simulink model "simulator_model"  (Simulink 8.4)
settings: Solver=ode45  StartTime=0.0  StopTime=inf  RelTol=1e-3
values from neighbouring files (symbols this model uses):
  beaver_b = 14.63    [asbdhc2_init.mat]
  beaver_c = 1.5875    [asbdhc2_init.mat]
  beaver_init_p = 0    [asbdhc2_init.mat]
  beaver_init_pitch = 0.13029612885    [asbdhc2_init.mat]
  beaver_init_q = 0    [asbdhc2_init.mat]
  beaver_init_r = 0    [asbdhc2_init.mat]
  beaver_init_roll = 0    [asbdhc2_init.mat]
  beaver_mass = 2288.231    [asbdhc2_init.mat]
  Cl0 = 0.000591    [asbdhc2_init.mat]
  Cl_alpha2_dpt = -0.01406    [asbdhc2_init.mat]
  Cl_beta = -0.0618    [asbdhc2_init.mat]
  Cl_da = -0.09917    [asbdhc2_init.mat]
  Cl_da_alpha = -0.08269    [asbdhc2_init.mat]
  Cl_dr = 0.006934    [asbdhc2_init.mat]
  Cl_p = -0.5045    [asbdhc2_init.mat]
  Cl_r = 0.1695    [asbdhc2_init.mat]
  Cm0 = 0.09448    [asbdhc2_init.mat]
  Cm_alpha = -0.6028    [asbdhc2_init.mat]
  Cm_alpha2 = -2.14    [asbdhc2_init.mat]
  Cm_beta2 = 0.6921    [asbdhc2_init.mat]
  Cm_de = -1.921    [asbdhc2_init.mat]
  Cm_df = 0.4072    [asbdhc2_init.mat]
  Cm_dpt = -0.07895    [asbdhc2_init.mat]
  Cm_q = -15.56    [asbdhc2_init.mat]
  Cm_r = -0.3118    [asbdhc2_init.mat]
  Cn0 = -0.003117    [asbdhc2_init.mat]
  Cn_beta = 0.006719    [asbdhc2_init.mat]
  Cn_beta3 = 0.1373    [asbdhc2_init.mat]
  Cn_da = -0.003872    [asbdhc2_init.mat]
  Cn_dpt3 = -0.003026    [asbdhc2_init.mat]
  Cn_dr = -0.08265    [asbdhc2_init.mat]
  Cn_p = -0.1585    [asbdhc2_init.mat]
  Cn_q = 0.1595    [asbdhc2_init.mat]
  Cn_r = -0.1112    [asbdhc2_init.mat]
  Cx0 = -0.03554    [asbdhc2_init.mat]
  Cx_alpha = 0.00292    [asbdhc2_init.mat]
  Cx_alpha2 = 5.459    [asbdhc2_init.mat]
  Cx_alpha3 = -5.162    [asbdhc2_init.mat]
  Cx_df = -0.09447    [asbdhc2_init.mat]
  Cx_df_alpha = 1.106    [asbdhc2_init.mat]
  Cx_dpt = 0.1161    [asbdhc2_init.mat]
  Cx_dpt2_alpha = 0.1453    [asbdhc2_init.mat]
  Cx_dr = 0.03412    [asbdhc2_init.mat]
  Cx_q = -0.6748    [asbdhc2_init.mat]
  Cy0 = -0.002226    [asbdhc2_init.mat]
  Cy_beta = -0.7678    [asbdhc2_init.mat]
  Cy_da = -0.02956    [asbdhc2_init.mat]
  Cy_dr = 0.1158    [asbdhc2_init.mat]
  Cy_dr_alpha = 0.5238    [asbdhc2_init.mat]
  Cy_p = -0.124    [asbdhc2_init.mat]
  Cy_r = 0.3666    [asbdhc2_init.mat]
  Cz0 = -0.05504    [asbdhc2_init.mat]
  Cz_alpha = -5.578    [asbdhc2_init.mat]
  Cz_alpha3 = 3.442    [asbdhc2_init.mat]
  Cz_de = -0.398    [asbdhc2_init.mat]
  Cz_de_beta = -15.93    [asbdhc2_init.mat]
  Cz_df = -1.377    [asbdhc2_init.mat]
  Cz_df_alpha = -1.261    [asbdhc2_init.mat]
  Cz_dpt = -0.1563    [asbdhc2_init.mat]
  Cz_q = -2.988    [asbdhc2_init.mat]
  uaero0 = [-0.0317656979071 -0.0320210159663 -0.0365180369264 0]    [asbdhc2_init.mat]
undefined symbols (not defined in the file or in its folder): Earth, F, Light, MIL, sigbuilder_block, WGS84
libraries: vrlib x8, aerolibtransform2 x5, aerolibconvert2 x4, aerolibwind2 x3, aerolibfltsims x2, aerolibasang x2, aerolibanimutils x1, aerolibatmos2 x1, aerolibgravity2 x1, aerolib6dof2 x1, aerolibadyn x1
settings Model: Creator=AMANALLAH  LastModifiedBy=AMANALLAH
settings DataIOCC: SignalLoggingSaveFormat=Dataset
settings OptimizationCC: ExpressionDepthLimit=128
settings DebuggingCC: UnderspecifiedInitializationDetection=Simplified  MergeDetectMultiDrivingBlocksExec=error  FcnCallInpInsideContextMsg=EnableAllAsError  StateNameClashWarn=none
settings GRTTargetCC: CombineOutputUpdateFcns=on  GRTInterface=off

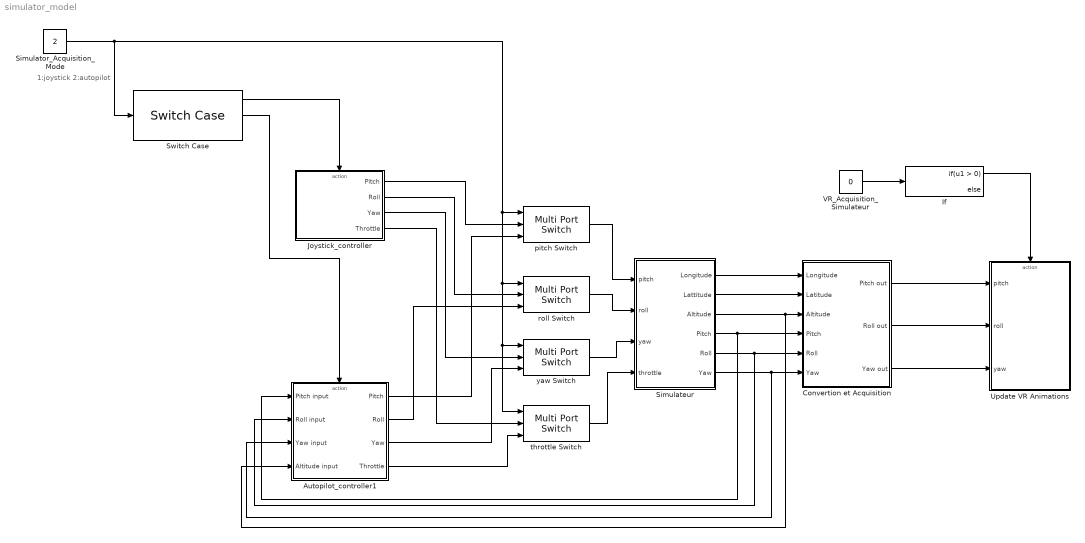
== system simulator_model ==
  note: 1:joystick
      | 2:autopilot
  Autopilot_controller1 : Subsystem  TreatAsAtomicUnit=on
  Convertion et Acquisition : Subsystem
  If : If  SampleTime=0.1
  Joystick_controller : Subsystem  TreatAsAtomicUnit=on
  Simulateur : Subsystem
  Simulator_Acquisition_Mode : Constant  Value=2
  Switch Case : SwitchCase  CaseConditions={1,2}  SampleTime=1/30
  Update VR Animations : Subsystem  TreatAsAtomicUnit=on
  VR_Acquisition_Simulateur : Constant  Value=0
  pitch Switch : MultiPortSwitch  Inputs=2
  roll Switch : MultiPortSwitch  Inputs=2
  throttle Switch : MultiPortSwitch  Inputs=2
  yaw Switch : MultiPortSwitch  Inputs=2
  wires:
  Simulateur/1(Longitude) -> Convertion et Acquisition/1(Longitude)
  Simulateur/2(Lattitude) -> Convertion et Acquisition/2(Latitude)
  Simulateur/3(Altitude) -> Autopilot_controller1/4(Altitude input), Convertion et Acquisition/3(Altitude)
  Simulateur/4(Pitch) -> Autopilot_controller1/1(Pitch input), Convertion et Acquisition/4(Pitch)
  Simulateur/5(Roll) -> Autopilot_controller1/2(Roll input), Convertion et Acquisition/5(Roll)
  Simulateur/6(Yaw) -> Autopilot_controller1/3(Yaw input), Convertion et Acquisition/6(Yaw)
  Convertion et Acquisition/1(Pitch out) -> Update VR Animations/1(pitch)
  Convertion et Acquisition/2(Roll out) -> Update VR Animations/2(roll)
  Convertion et Acquisition/3(Yaw out) -> Update VR Animations/3(yaw)
  pitch Switch/1 -> Simulateur/1(pitch)
  roll Switch/1 -> Simulateur/2(roll)
  yaw Switch/1 -> Simulateur/3(yaw)
  throttle Switch/1 -> Simulateur/4(throttle)
  Autopilot_controller1/1(Pitch) -> pitch Switch/3
  Joystick_controller/1(Pitch) -> pitch Switch/2
  Autopilot_controller1/2(Roll) -> roll Switch/3
  Joystick_controller/2(Roll) -> roll Switch/2
  Joystick_controller/3(Yaw) -> yaw Switch/2
  Autopilot_controller1/3(Yaw) -> yaw Switch/3
  Joystick_controller/4(Throttle) -> throttle Switch/2
  Simulator_Acquisition_Mode/1 -> throttle Switch/1, yaw Switch/1, roll Switch/1, pitch Switch/1, Switch Case/1
  Switch Case/1 -> Joystick_controller/Action
  If/1 -> Update VR Animations/Action
  VR_Acquisition_Simulateur/1 -> If/1
  Autopilot_controller1/4(Throttle) -> throttle Switch/3
  Switch Case/2 -> Autopilot_controller1/Action

== system simulator_model/Autopilot_controller1 ==
  Pitch input : Inport
  Roll input : Inport  Port=2
  Yaw input : Inport  Port=3
  Altitude input : Inport  Port=4
  Action Port : ActionPort  ActionType=case
  Constant{,1..3} (4 alike) : Constant  Value=0
  Pitch : Outport
  Roll : Outport  Port=2
  Yaw : Outport  Port=3
  Throttle : Outport  Port=4
  wires:
  Constant/1 -> Pitch/1
  Constant1/1 -> Roll/1
  Constant2/1 -> Yaw/1
  Constant3/1 -> Throttle/1

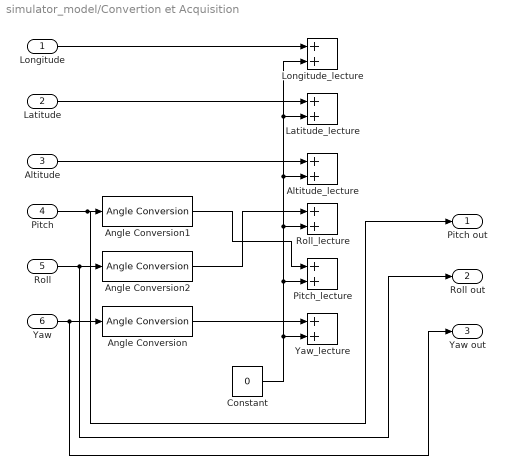
== system simulator_model/Convertion et Acquisition ==
  Longitude : Inport
  Latitude : Inport  Port=2
  Altitude : Inport  Port=3
  Pitch : Inport  Port=4
  Roll : Inport  Port=5
  Yaw : Inport  Port=6
  Altitude_lecture : Sum
  Angle Conversion : aerolibconvert2/Angle Conversion  IU=rad  OU=deg
  Angle Conversion1 : aerolibconvert2/Angle Conversion  IU=rad  OU=deg
  Angle Conversion2 : aerolibconvert2/Angle Conversion  IU=rad  OU=deg
  Constant : Constant  Value=0
  Latitude_lecture : Sum
  Longitude_lecture : Sum
  Pitch_lecture : Sum
  Roll_lecture : Sum
  Yaw_lecture : Sum
  Pitch out : Outport
  Roll out : Outport  Port=2
  Yaw out : Outport  Port=3
  wires:
  Altitude/1 -> Altitude_lecture/1
  Longitude/1 -> Longitude_lecture/1
  Latitude/1 -> Latitude_lecture/1
  Roll/1 -> Angle Conversion2/1, Roll out/1
  Pitch/1 -> Pitch out/1, Angle Conversion1/1
  Constant/1 -> Pitch_lecture/2, Roll_lecture/2, Altitude_lecture/2, Latitude_lecture/2, Longitude_lecture/2, Yaw_lecture/2
  Angle Conversion/1 -> Yaw_lecture/1
  Angle Conversion1/1 -> Pitch_lecture/1
  Angle Conversion2/1 -> Roll_lecture/1
  Yaw/1 -> Angle Conversion/1, Yaw out/1

== system simulator_model/Joystick_controller ==
  Action Port : ActionPort  ActionType=case
  Pilot Joystick : aerolibanimutils/Pilot Joystick  JoystickID=Joystick1  OutputConfiguration=FourAxis  SampleTime=1/30
  Pitch : Outport
  Roll : Outport  Port=2
  Yaw : Outport  Port=3
  Throttle : Outport  Port=4
  wires:
  Pilot Joystick/2 -> Pitch/1
  Pilot Joystick/1 -> Roll/1
  Pilot Joystick/3 -> Yaw/1
  Pilot Joystick/4 -> Throttle/1

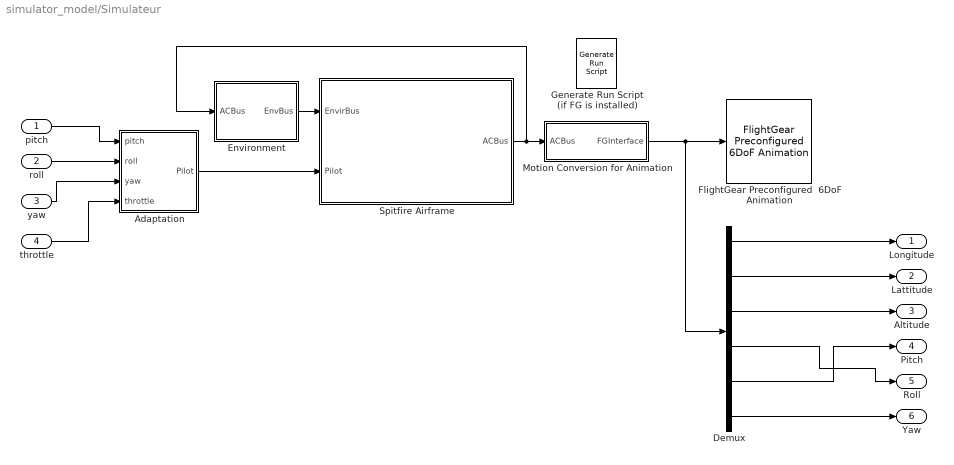
== system simulator_model/Simulateur ==
  pitch : Inport
  roll : Inport  Port=2
  yaw : Inport  Port=3
  throttle : Inport  Port=4
  "Adaptation " : Subsystem
  Demux : Demux  Outputs=6
  Environment : Subsystem
  FlightGear Preconfigured  6DoF Animation : aerolibfltsims/FlightGear Preconfigured 6DoF Animation  xFlightGearVersion=v3.0  DestinationIpAddress=127.0.0.1  DestinationPort=5502  SampleTime=1/30
  Generate Run Script (if FG is installed) : aerolibfltsims/Generate Run Script  OutputFileName=runfg.bat  FlightGearBaseDirectory=C:\Program Files\FlightGear  GeometryModelName=dhc2F  DestinationPort=5502  OriginAddress=127.0.0.1  OriginPort=5505  LocalAddress=127.0.0.1  AirportId=KSFO  RunwayId=10L  InitialAltitude=7224  InitialHeading=113  OffsetDistance=4.72  OffsetAzimuth=0  GenerateFile=off  Architecture=Default  dataFlow=Send
  Motion Conversion for Animation : Subsystem
      mask Display:
      | port_label('input',1,'ACBus')
      | port_label('output',1,'\lambda,L,h,\phi,\theta,\psi','texmode','on')
  Spitfire Airframe : Subsystem
      mask Display: image(imread([pwd,'\Ressources\images\spitfire.jpg']));
  Longitude : Outport
  Lattitude : Outport  Port=2
  Altitude : Outport  Port=3
  Pitch : Outport  Port=4
  Roll : Outport  Port=5
  Yaw : Outport  Port=6
  wires:
  Spitfire Airframe/1(ACBus) -> Motion Conversion for Animation/1(ACBus), Environment/1(ACBus)
  "Adaptation "/1(Pilot) -> Spitfire Airframe/2(Pilot)
  Environment/1(EnvBus) -> Spitfire Airframe/1(EnvirBus)
  Motion Conversion for Animation/1(FGInterface) -> Demux/1, FlightGear Preconfigured  6DoF Animation/1
  pitch/1 -> "Adaptation "/1(pitch)
  roll/1 -> "Adaptation "/2(roll)
  yaw/1 -> "Adaptation "/3(yaw)
  throttle/1 -> "Adaptation "/4(throttle)
  Demux/1 -> Longitude/1
  Demux/2 -> Lattitude/1
  Demux/3 -> Altitude/1
  Demux/4 -> Roll/1
  Demux/5 -> Pitch/1
  Demux/6 -> Yaw/1

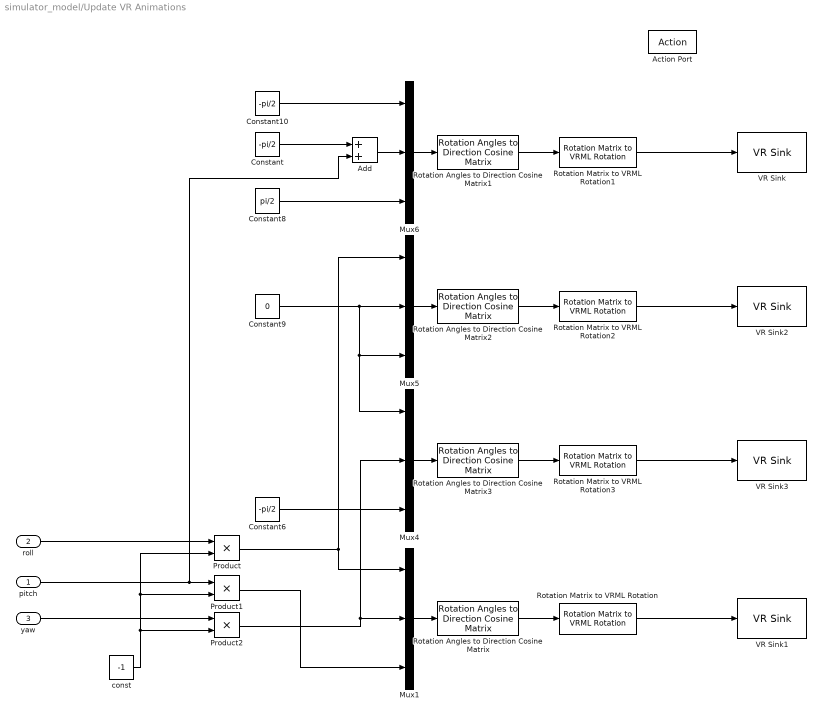
== system simulator_model/Update VR Animations ==
  pitch : Inport
  roll : Inport  Port=2
  yaw : Inport  Port=3
  Action Port : ActionPort  ActionType=then
  Add : Sum
  Constant : Constant  Value=-pi/2
  Constant10 : Constant  Value=-pi/2
  Constant6 : Constant  Value=-pi/2
  Constant8 : Constant  Value=pi/2
  Constant9 : Constant  Value=0
  Mux{1,4..6} (4 alike) : Mux  Inputs=3
  Product : Product
  Product1 : Product
  Product2 : Product
  Rotation Angles to Direction Cosine Matrix{,1..3} (4 alike) : aerolibtransform2/Rotation Angles to Direction Cosine Matrix  rotationOrder=ZYX
  Rotation Matrix to VRML Rotation{,1..3} (4 alike) : vrlib/Utilities/Rotation Matrix to VRML Rotation  maxzero=1e-12
  VR Sink : vrlib/VR Sink  InstantiateOnLoad=on  SampleTime=0.1  ViewEnable=on  RemoteChange=off  RemoteView=off  FieldsWritten=Airplane.rotation.4.1.1.double  WorldFileName=spitfire_3d_pitch.WRL  AutoView=off  VideoDimensions=[]  AllowVariableSize=off
  VR Sink1 : vrlib/VR Sink  InstantiateOnLoad=on  SampleTime=0.1  ViewEnable=on  RemoteChange=off  RemoteView=off  FieldsWritten=Airplane.rotation.4.1.1.double  WorldFileName=spitfire_3d.WRL  AutoView=off  VideoDimensions=[]  AllowVariableSize=off
  VR Sink2 : vrlib/VR Sink  InstantiateOnLoad=on  SampleTime=0.1  ViewEnable=on  RemoteChange=off  RemoteView=off  FieldsWritten=Airplane.rotation.4.1.1.double  WorldFileName=spitfire_3d_roll.WRL  AutoView=off  VideoDimensions=[]  AllowVariableSize=off
  VR Sink3 : vrlib/VR Sink  InstantiateOnLoad=on  SampleTime=0.1  ViewEnable=on  RemoteChange=off  RemoteView=off  FieldsWritten=Airplane.rotation.4.1.1.double  WorldFileName=spitfire_3d_yaw.WRL  AutoView=off  VideoDimensions=[]  AllowVariableSize=off
  const : Constant  Value=-1
  wires:
  Rotation Matrix to VRML Rotation/1 -> VR Sink1/1
  Rotation Angles to Direction Cosine Matrix/1 -> Rotation Matrix to VRML Rotation/1
  Mux1/1 -> Rotation Angles to Direction Cosine Matrix/1
  Mux6/1 -> Rotation Angles to Direction Cosine Matrix1/1
  Rotation Angles to Direction Cosine Matrix1/1 -> Rotation Matrix to VRML Rotation1/1
  Rotation Matrix to VRML Rotation1/1 -> VR Sink/1
  Mux5/1 -> Rotation Angles to Direction Cosine Matrix2/1
  Rotation Angles to Direction Cosine Matrix2/1 -> Rotation Matrix to VRML Rotation2/1
  Rotation Matrix to VRML Rotation2/1 -> VR Sink2/1
  Mux4/1 -> Rotation Angles to Direction Cosine Matrix3/1
  Rotation Angles to Direction Cosine Matrix3/1 -> Rotation Matrix to VRML Rotation3/1
  Rotation Matrix to VRML Rotation3/1 -> VR Sink3/1
  Constant9/1 -> Mux4/1, Mux5/3, Mux5/2
  Constant6/1 -> Mux4/3
  Constant10/1 -> Mux6/1
  Constant8/1 -> Mux6/3
  Constant/1 -> Add/1
  Add/1 -> Mux6/2
  Product/1 -> Mux1/1, Mux5/1
  Product2/1 -> Mux4/2, Mux1/2
  Product1/1 -> Mux1/3
  roll/1 -> Product/1
  pitch/1 -> Product1/1, Add/2
  yaw/1 -> Product2/1
  const/1 -> Product/2, Product1/2, Product2/2

== system simulator_model/Simulateur/Adaptation  ==
  pitch : Inport
  roll : Inport  Port=2
  yaw : Inport  Port=3
  throttle : Inport  Port=4
  Bus Creator : BusCreator  Inputs=2
  Flap : Subsystem  Tag=STV Subsys  LoadFcn=sigbuilder_block('load');  StartFcn=sigbuilder_block('start');  StopFcn=sigbuilder_block('stop');  ClipboardFcn=sigbuilder_block('clipboard');  mask(Sigbuilder block){}
      mask help: Sigbuilder GUI
      mask init:
      | if ~strcmp(get_param(bdroot(gcb),'SimulationStatus'),'stopped') tuvar = sigbuilder_block('maskInit'); end
      settings: CopyFcn=sigbuilder_block('copy');  DeleteFcn=sigbuilder_block('delete');  ModelCloseFcn=sigbuilder_block('modelClose');  PreSaveFcn=sigbuilder_block('preSave');  PauseFcn=sigbuilder_block('pause')  ContinueFcn=sigbuilder_block('continue')  NameChangeFcn=sigbuilder_block('namechange');  OpenFcn=sigbuilder_block('open',[127.2 252 511.2 271.2 ]);  CloseFcn=sigbuilder_block('close');
      mask Display: plot(0,0,100,100,[10,10,40,40,10],[80,20,20,80,80],[40,10],[50,50], [40,27,10],[65,72,56],[40,25,25,10],[28,28,43,43]);
  Input Signal  Conditioning : Subsystem
  Mux2 : Mux  Inputs=3
  Rate Transition1 : RateTransition  OutPortSampleTime=0
  Rate Transition2 : RateTransition  OutPortSampleTime=0
  Pilot : Outport
  wires:
  Flap/1(Flap) -> Input Signal  Conditioning/3(Flap)
  Rate Transition1/1 -> Input Signal  Conditioning/1(Stick / Throt)
  Rate Transition2/1 -> Input Signal  Conditioning/2(Rudder)
  Input Signal  Conditioning/1(uaero) -> Bus Creator/1  "uaero"
  Input Signal  Conditioning/2(uprop) -> Bus Creator/2  "uprop"
  Bus Creator/1 -> Pilot/1
  Mux2/1 -> Rate Transition1/1
  roll/1 -> Mux2/1
  yaw/1 -> Rate Transition2/1
  throttle/1 -> Mux2/3
  pitch/1 -> Mux2/2

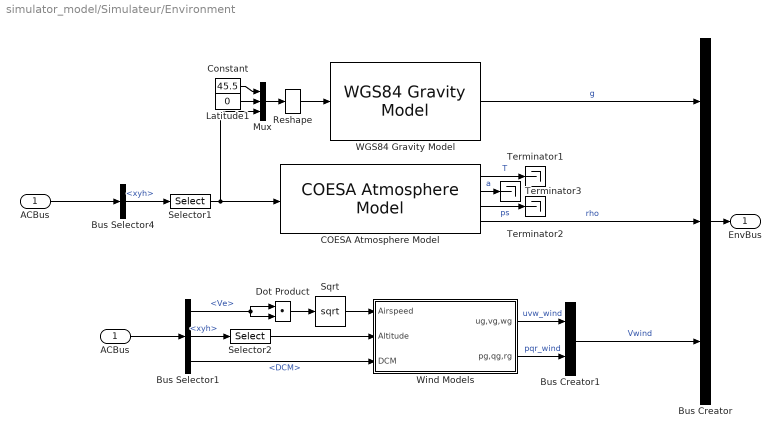
== system simulator_model/Simulateur/Environment ==
  ACBus : Inport
  "ACBus " : InportShadow
  Bus Creator : BusCreator  Inputs=3
  Bus Creator1 : BusCreator  Inputs=2
  Bus Selector1 : BusSelector  OutputSignals=Ve,xyh,DCM
  Bus Selector4 : BusSelector  OutputSignals=xyh
  COESA Atmosphere Model : aerolibatmos2/COESA Atmosphere Model  units=Metric (MKS)  spec=1976 COESA-extended U.S. Standard Atmosphere  model=Profile  profile_var=High temperature  profile_percent=1%  profile_alt=5 km (16404 ft)  envelope_var=High temperature  envelope_percent=1%  action=Warning
  Constant : Constant  Value=45.5
  Dot Product : DotProduct  InputSameDT=on  OutDataTypeStr=Inherit: Inherit via internal rule
  Latitude1 : Constant  Value=0
  Mux : Mux  Inputs=3
  Reshape : Reshape  OutputDimensionality=Row vector (2-D)
  Selector1 : Selector  IndexMode=Zero-based  InputPortWidth=3  Indices=2
  Selector2 : Selector  IndexMode=Zero-based  InputPortWidth=3  Indices=2
  Sqrt : Sqrt  SaturateOnIntegerOverflow=on
  Terminator1 : Terminator
  Terminator2 : Terminator
  Terminator3 : Terminator
  "WGS84 Gravity Model " : aerolibgravity2/WGS84 Gravity Model   model=WGS84 Taylor Series  units=Metric (MKS)  no_atmos=on  precessing=on  jd_loc=off  month=October  day=10  year=2004  no_centrifugal=on  action=None
  Wind Models : Subsystem
  EnvBus : Outport
  wires:
  COESA Atmosphere Model/4 -> Bus Creator/2  "rho"
  COESA Atmosphere Model/1 -> Terminator1/1  "T"
  COESA Atmosphere Model/3 -> Terminator2/1  "ps"
  COESA Atmosphere Model/2 -> Terminator3/1  "a"
  Selector1/1 -> COESA Atmosphere Model/1, Mux/3
  Bus Selector1/3 -> Wind Models/3(DCM)  "<DCM>"
  Wind Models/2(pg,qg,rg) -> Bus Creator1/2  "pqr_wind"
  Wind Models/1(ug,vg,wg) -> Bus Creator1/1  "uvw_wind"
  Bus Creator1/1 -> Bus Creator/3  "Vwind"
  Dot Product/1 -> Sqrt/1
  Sqrt/1 -> Wind Models/1(Airspeed)
  Bus Creator/1 -> EnvBus/1
  ACBus/1 -> Bus Selector4/1
  Bus Selector4/1 -> Selector1/1  "<xyh>"
  "ACBus "/1 -> Bus Selector1/1
  Bus Selector1/2 -> Selector2/1  "<xyh>"
  Selector2/1 -> Wind Models/2(Altitude)
  Bus Selector1/1 -> Dot Product/1, Dot Product/2  "<Ve>"
  Constant/1 -> Mux/1
  Latitude1/1 -> Mux/2
  Mux/1 -> Reshape/1
  "WGS84 Gravity Model "/1 -> Bus Creator/1  "g"
  Reshape/1 -> "WGS84 Gravity Model "/1

== system simulator_model/Simulateur/Motion Conversion for Animation ==
  ACBus : Inport
  Bus Selector : BusSelector  OutputSignals=phi_theta_psi
  Bus Selector1 : BusSelector  OutputSignals=Xe  OutputAsBus=on
  Constant : Constant  Value=0
  Flat Earth to LLA : aerolibtransform2/Flat Earth to LLA  units=Metric (MKS)  ptype=Earth (WGS84)  F=1/298.257223563  R=6378137  LL0=[37.6272 -122.3896]  psi=0
  Mux : Mux  Inputs=2
  Mux1 : Mux  Inputs=2
  Selector : Selector  IndexMode=Zero-based  InputPortWidth=2  Indices=[1 0]
  FGInterface : Outport
  wires:
  Mux1/1 -> FGInterface/1
  Constant/1 -> Flat Earth to LLA/2
  Bus Selector/1 -> Mux1/2  "<phi_theta_psi>"
  Mux/1 -> Mux1/1
  Flat Earth to LLA/2 -> Mux/2
  Flat Earth to LLA/1 -> Selector/1
  Bus Selector1/1 -> Flat Earth to LLA/1
  ACBus/1 -> Bus Selector/1, Bus Selector1/1
  Selector/1 -> Mux/1

== system simulator_model/Simulateur/Spitfire Airframe ==
  EnvirBus : Inport
  Pilot : Inport  Port=2
  Aircraft Dynamics : Subsystem
  Calculate Parameters : Subsystem
  ACBus : Outport
  wires:
  Pilot/1 -> Aircraft Dynamics/1(Pilot)
  Aircraft Dynamics/1(AC Bus) -> ACBus/1, Calculate Parameters/2(ACBus)
  EnvirBus/1 -> Aircraft Dynamics/2(EnvirBus), Calculate Parameters/1(EnvirBus)
  Calculate Parameters/1(FltParams) -> Aircraft Dynamics/3(FltParams)

== system simulator_model/Simulateur/Adaptation /Flap ==
  Demux : Demux  Tag=STV Demux  Outputs=1
  FromWs : FromWorkspace  Tag=STV FromWs  VariableName=tuvar  SampleTime=0  OutputAfterFinalValue=Holding final value  SigBuilderData=DataTag0  VnvData=DataTag1
      SigBuilderData=|
      | dataSet.timeRange = [0 300]
      | dataSet.name = 'Group 1'
      | sbobj.Groups.Name = 'Group 1'
      | sbobj.Groups.Signals.Name = 'Flap'
      | sbobj.Groups.Signals.XData = [0 4 6 300]
      | sbobj.Groups.Signals.YData = [0 0 0 0]
      | sbobj.Groups.TimeRange = [0 300]
  Flap : Outport  Tag=STV Outport
  wires:
  Demux/1 -> Flap/1
  FromWs/1 -> Demux/1

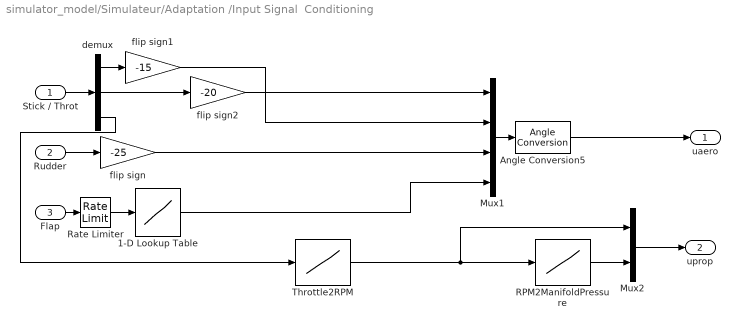
== system simulator_model/Simulateur/Adaptation /Input Signal  Conditioning ==
  Stick / Throt : Inport
  Rudder : Inport  Port=2
  Flap : Inport  Port=3
  1-D Lookup Table : Lookup_n-D  NumberOfTableDimensions=1  BreakpointsForDimension1=[0:3]  Table=[0 4 10 20]  SaturateOnIntegerOverflow=on  InputSameDT=on
  Angle Conversion5 : aerolibconvert2/Angle Conversion  IU=deg  OU=rad
  Mux1 : Mux
  Mux2 : Mux  Inputs=2
  RPM2ManifoldPressure : Lookup_n-D  NumberOfTableDimensions=1  BreakpointsForDimension1=[0 1800 2300]  IndexSearchMethod=Linear search  BeginIndexSearchUsingPreviousIndexResult=on  Table=[0 22.5735 26]  ExtrapMethod=Clip  InputSameDT=on
  Rate Limiter : RateLimiter  RisingSlewLimit=0.5  FallingSlewLimit=-0.5
  Throttle2RPM : Lookup_n-D  NumberOfTableDimensions=1  BreakpointsForDimension1=(1/6)*(3+([-3:3]))  IndexSearchMethod=Linear search  BeginIndexSearchUsingPreviousIndexResult=on  Table=((1+tanh([-3:3]))/(1+tanh(2.65))-0.0025)*2300  ExtrapMethod=Clip  InputSameDT=on
  demux : Demux  Outputs=3
  flip sign : Gain  Gain=-25  SaturateOnIntegerOverflow=on  OutDataTypeStr=Inherit: Same as input  ParamDataTypeStr=Inherit: Same as input
  flip sign1 : Gain  Gain=-15  SaturateOnIntegerOverflow=on  OutDataTypeStr=Inherit: Same as input  ParamDataTypeStr=Inherit: Same as input
  flip sign2 : Gain  Gain=-20  SaturateOnIntegerOverflow=on  OutDataTypeStr=Inherit: Same as input  ParamDataTypeStr=Inherit: Same as input
  uaero : Outport
  uprop : Outport  Port=2
  wires:
  demux/3 -> Throttle2RPM/1
  Flap/1 -> Rate Limiter/1
  Rate Limiter/1 -> 1-D Lookup Table/1
  Stick / Throt/1 -> demux/1
  Rudder/1 -> flip sign/1
  1-D Lookup Table/1 -> Mux1/4
  demux/1 -> flip sign1/1
  demux/2 -> flip sign2/1
  Mux1/1 -> Angle Conversion5/1
  Angle Conversion5/1 -> uaero/1
  RPM2ManifoldPressure/1 -> Mux2/2
  Mux2/1 -> uprop/1
  flip sign/1 -> Mux1/3
  Throttle2RPM/1 -> Mux2/1, RPM2ManifoldPressure/1
  flip sign1/1 -> Mux1/2
  flip sign2/1 -> Mux1/1

== system simulator_model/Simulateur/Environment/Wind Models ==
  Airspeed : Inport
  Altitude : Inport  Port=2
  DCM : Inport  Port=3
  "DCM " : InportShadow  Port=3
  Discrete Wind Gust Model : aerolibwind2/Discrete Wind Gust Model  units=Metric (MKS)  Gx=off  Gy=off  Gz=off  t_0=20  d_m=[120 120 80]  v_m=[3.5 3.5 3.0]
  Dryden Wind Turbulence Model  (Continuous (+q -r)) : aerolibwind2/Dryden Wind Turbulence Model  (Continuous (+q -r))  units=Metric (MKS)  spec=MIL-F-8785C  model=Continuous Dryden (+q -r)  W20=5  Wdeg=0  TurbProb=10^-2 - Light  L_high=533.4  Wingspan=4  ts=0.1  Seed=[23341 23342 23343 23344]  T_on=off
  Sum : Sum  Inputs=+++  SaturateOnIntegerOverflow=on  InputSameDT=on  OutDataTypeStr=Inherit: Same as first input
  Wind Shear Model : aerolibwind2/Wind Shear Model  units=Metric (MKS)  phase=Category C - Terminal Flight Phase  W_20=0  Wdeg=0
  ug,vg,wg : Outport
  pg,qg,rg : Outport  Port=2
  wires:
  "DCM "/1 -> Dryden Wind Turbulence Model  (Continuous (+q -r))/3
  Wind Shear Model/1 -> Sum/1
  Dryden Wind Turbulence Model  (Continuous (+q -r))/1 -> Sum/2
  Discrete Wind Gust Model/1 -> Sum/3
  Sum/1 -> ug,vg,wg/1
  DCM/1 -> Wind Shear Model/2
  Airspeed/1 -> Dryden Wind Turbulence Model  (Continuous (+q -r))/2, Discrete Wind Gust Model/1
  Dryden Wind Turbulence Model  (Continuous (+q -r))/2 -> pg,qg,rg/1
  Altitude/1 -> Dryden Wind Turbulence Model  (Continuous (+q -r))/1, Wind Shear Model/1

== system simulator_model/Simulateur/Spitfire Airframe/Aircraft Dynamics ==
  Pilot : Inport
  EnvirBus : Inport  Port=2
  FltParams : Inport  Port=3
  6DOF (Quaternion) : aerolib6dof2/6DOF (Euler Angles)  units=Metric (MKS)  mtype=Fixed  rep=Quaternion  xme_0=xme_0  Vm_0=[44.54 2.714 5.836]  eul_0=[beaver_init_roll, beaver_init_pitch, 113/180*pi]  pm_0=[beaver_init_p, beaver_init_q, beaver_init_r]  mass_0=beaver_mass  mass_e=0  mass_f=0  inertia="[5.787969e3  0 1.1764e2; 0 6.92893e3 0; -1.1764e2 0 1.1578329e4]"  inertia_e=eye(3)  inertia_f=eye(3)  k_quat=1.0  vre_flag=on
  Bus Creator : BusCreator  Inputs=8
  Hdot : Gain  Gain=-1  SaturateOnIntegerOverflow=on  OutDataTypeStr=Inherit: Same as input  ParamDataTypeStr=Inherit: Same as input
  Selector1 : Selector  IndexMode=Zero-based  InputPortWidth=3  Indices=2
  Terminator : Terminator
  Terminator1 : Terminator
  Total Forces  and Moments : Subsystem
  xyH : Gain  Gain=[1 1 -1]  SaturateOnIntegerOverflow=on  OutDataTypeStr=Inherit: Same as input  ParamDataTypeStr=Inherit: Same as input
  AC Bus : Outport
  wires:
  6DOF (Quaternion)/4 -> Bus Creator/6, Total Forces  and Moments/3(DCM)  "DCM"
  6DOF (Quaternion)/3 -> Bus Creator/5  "phi_theta_psi"
  6DOF (Quaternion)/2 -> xyH/1, Bus Creator/3  "Xe"
  6DOF (Quaternion)/5 -> Bus Creator/7  "Vbody"
  6DOF (Quaternion)/7 -> Terminator/1
  6DOF (Quaternion)/1 -> Selector1/1, Bus Creator/2  "Ve"
  Pilot/1 -> Total Forces  and Moments/2(Pilot)
  Selector1/1 -> Hdot/1
  Total Forces  and Moments/1(Total Force) -> 6DOF (Quaternion)/1
  Total Forces  and Moments/2(Total Moment) -> 6DOF (Quaternion)/2
  xyH/1 -> Bus Creator/4  "xyh"
  Hdot/1 -> Bus Creator/1  "Hdot"
  6DOF (Quaternion)/8 -> Terminator1/1
  Bus Creator/1 -> AC Bus/1
  EnvirBus/1 -> Total Forces  and Moments/1(EnvirBus)
  6DOF (Quaternion)/6 -> Bus Creator/8  "pqr"
  FltParams/1 -> Total Forces  and Moments/4(FltParams)

== system simulator_model/Simulateur/Spitfire Airframe/Calculate Parameters ==
  EnvirBus : Inport
  ACBus : Inport  Port=2
  "ACBus " : InportShadow  Port=2
  Bus Creator : BusCreator  Inputs=5
  Bus Selector1 : BusSelector  OutputSignals=rho
  Bus Selector2 : BusSelector  OutputSignals=Vbody
  Bus Selector3 : BusSelector  OutputSignals=pqr,Ve
  Bus Selector4 : BusSelector  OutputSignals=Vwind.uvw_wind,Vwind.pqr_wind
  Dynamic Pressure : aerolibasang/Dynamic Pressure
  "Incidence, Sideslip, & Airspeed" : aerolibasang/Incidence, Sideslip, & Airspeed
  Sum2 : Sum  Inputs=|++  SaturateOnIntegerOverflow=on  InputSameDT=on  OutDataTypeStr=Inherit: Same as first input
  Sum4 : Sum  Inputs=+-|  SaturateOnIntegerOverflow=on  InputSameDT=on  OutDataTypeStr=Inherit: Same as first input
  FltParams : Outport
  wires:
  "ACBus "/1 -> Bus Selector2/1
  Bus Creator/1 -> FltParams/1
  Bus Selector3/1 -> Sum2/2  "<pqr>"
  ACBus/1 -> Bus Selector3/1
  Bus Selector1/1 -> Dynamic Pressure/2  "<rho>"
  EnvirBus/1 -> Bus Selector1/1, Bus Selector4/1
  Dynamic Pressure/1 -> Bus Creator/5  "Qdyn"
  Bus Selector3/2 -> Dynamic Pressure/1  "<Ve>"
  Bus Selector4/2 -> Sum2/1  "<pqr_wind>"
  Sum4/1 -> "Incidence, Sideslip, & Airspeed"/1
  "Incidence, Sideslip, & Airspeed"/1 -> Bus Creator/1  "alpha"
  "Incidence, Sideslip, & Airspeed"/2 -> Bus Creator/2  "beta"
  "Incidence, Sideslip, & Airspeed"/3 -> Bus Creator/3  "V"
  Bus Selector2/1 -> Sum4/1  "<Vbody>"
  Bus Selector4/1 -> Sum4/2  "<uvw_wind>"
  Sum2/1 -> Bus Creator/4  "pqr_tot"

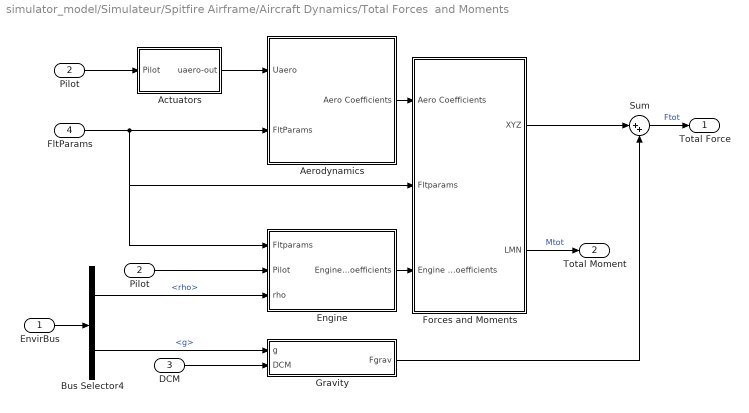
== system simulator_model/Simulateur/Spitfire Airframe/Aircraft Dynamics/Total Forces  and Moments ==
  EnvirBus : Inport
  Pilot : Inport  Port=2
  DCM : Inport  Port=3
  FltParams : Inport  Port=4
  Actuators : Subsystem
  Aerodynamics : Subsystem
  Bus Selector4 : BusSelector  OutputSignals=rho,g
  "Engine " : Subsystem
  Forces and Moments : Subsystem
  "Gravity " : Subsystem
  "Pilot " : InportShadow  Port=2
  Sum : Sum  Inputs=|++  SaturateOnIntegerOverflow=on  InputSameDT=on  OutDataTypeStr=Inherit: Same as first input
  Total Force : Outport
  Total Moment : Outport  Port=2
  wires:
  Forces and Moments/1(XYZ) -> Sum/1
  "Engine "/1(Engine Coefficients) -> Forces and Moments/3(Engine Coefficients)
  "Gravity "/1(Fgrav) -> Sum/2
  Aerodynamics/1(Aero Coefficients) -> Forces and Moments/1(Aero Coefficients)
  Pilot/1 -> Actuators/1(Pilot)
  Bus Selector4/1 -> "Engine "/3(rho)  "<rho>"
  DCM/1 -> "Gravity "/2(DCM)
  Bus Selector4/2 -> "Gravity "/1(g)  "<g>"
  Sum/1 -> Total Force/1  "Ftot"
  Forces and Moments/2(LMN) -> Total Moment/1  "Mtot"
  "Pilot "/1 -> "Engine "/2(Pilot)
  FltParams/1 -> "Engine "/1(Fltparams), Forces and Moments/2(Fltparams), Aerodynamics/2(FltParams)
  Actuators/1(uaero-out) -> Aerodynamics/1(Uaero)
  EnvirBus/1 -> Bus Selector4/1

== system simulator_model/Simulateur/Spitfire Airframe/Aircraft Dynamics/Total Forces  and Moments/Actuators ==
  Pilot : Inport
  Bus Selector2 : BusSelector  OutputSignals=uaero
  Demux : Demux
  Initial inputs for aero : Constant  Value=uaero0
  Mux : Mux
  Sum1 : Sum  Inputs=++|  SaturateOnIntegerOverflow=on  InputSameDT=on  OutDataTypeStr=Inherit: Same as first input
  uaero-out : Outport
  wires:
  Pilot/1 -> Bus Selector2/1
  Initial inputs for aero/1 -> Sum1/1
  Sum1/1 -> uaero-out/1
  Bus Selector2/1 -> Demux/1  "<uaero>"
  Demux/4 -> Mux/4
  Demux/1 -> Mux/1
  Demux/2 -> Mux/2
  Demux/3 -> Mux/3
  Mux/1 -> Sum1/2

== system simulator_model/Simulateur/Spitfire Airframe/Aircraft Dynamics/Total Forces  and Moments/Aerodynamics ==
  Uaero : Inport
  FltParams : Inport  Port=2
  Actuator Increments : Subsystem
  Body Rate Damping : Subsystem
  Bus Selector1 : BusSelector  OutputSignals=alpha,beta
  Bus Selector2 : BusSelector  OutputSignals=V,pqr_tot
  Datum Coefficients : Subsystem
  Sum : Sum  Inputs=+++  SaturateOnIntegerOverflow=on
  Aero Coefficients : Outport
  wires:
  Bus Selector1/2 -> Actuator Increments/2(beta), Datum Coefficients/2(beta)  "<beta>"
  Sum/1 -> Aero Coefficients/1
  Body Rate Damping/1(Coefficients) -> Sum/3
  Datum Coefficients/1(Coefficients) -> Sum/1
  Actuator Increments/1(Coefficients) -> Sum/2
  Bus Selector2/1 -> Body Rate Damping/1(V)  "<V>"
  Bus Selector2/2 -> Body Rate Damping/2(p,q,r)  "<pqr_tot>"
  Uaero/1 -> Actuator Increments/3(Actuator Deflections)
  Bus Selector1/1 -> Actuator Increments/1(alpha), Datum Coefficients/1(alpha)  "<alpha>"
  FltParams/1 -> Bus Selector1/1, Bus Selector2/1

== system simulator_model/Simulateur/Spitfire Airframe/Aircraft Dynamics/Total Forces  and Moments/Engine  ==
  Fltparams : Inport
  Pilot : Inport  Port=2
  rho : Inport  Port=3
  Bus Selector4 : BusSelector  OutputSignals=V,alpha
  eng : Subsystem
  pow : Subsystem
  Engine Coefficients : Outport
  wires:
  Bus Selector4/1 -> pow/3(V)  "<V>"
  rho/1 -> pow/1(rho)
  Bus Selector4/2 -> eng/2(alpha)  "<alpha>"
  eng/1(Cprop) -> Engine Coefficients/1
  Pilot/1 -> pow/2(Pilot)
  pow/1(dpt) -> eng/1(dpt)
  Fltparams/1 -> Bus Selector4/1

== system simulator_model/Simulateur/Spitfire Airframe/Aircraft Dynamics/Total Forces  and Moments/Forces and Moments ==
  Aero Coefficients : Inport
  Fltparams : Inport  Port=2
  Engine Coefficients : Inport  Port=3
  Aerodynamic Forces and Moments : aerolibadyn/Aerodynamic Forces and Moments   inputAxes=Body  outputForceAxes=Body  outputMomentAxes=Body  S=beaver_S  b=beaver_b  cbar=beaver_c
  Bus Selector4 : BusSelector  OutputSignals=Qdyn
  Sum : Sum  Inputs=++|  SaturateOnIntegerOverflow=on  InputSameDT=on  OutDataTypeStr=Inherit: Same as first input
  neglect center of gravity  and center of pressure effects : Constant  Value=[0 0 0]
  XYZ : Outport
  LMN : Outport  Port=2
  wires:
  Sum/1 -> Aerodynamic Forces and Moments/1
  Aero Coefficients/1 -> Sum/2
  Engine Coefficients/1 -> Sum/1
  Aerodynamic Forces and Moments/2 -> LMN/1
  Fltparams/1 -> Bus Selector4/1
  Aerodynamic Forces and Moments/1 -> XYZ/1
  neglect center of gravity  and center of pressure effects/1 -> Aerodynamic Forces and Moments/3, Aerodynamic Forces and Moments/4
  Bus Selector4/1 -> Aerodynamic Forces and Moments/2  "<Qdyn>"

== system simulator_model/Simulateur/Spitfire Airframe/Aircraft Dynamics/Total Forces  and Moments/Gravity  ==
  g : Inport
  DCM : Inport  Port=2
  Gravity in Earth Axes : Gain  Gain=beaver_mass  SaturateOnIntegerOverflow=on  OutDataTypeStr=Inherit: Same as input  ParamDataTypeStr=Inherit: Same as input
  Inertial to Body : Product  Multiplication=Matrix(*)  SaturateOnIntegerOverflow=on  InputSameDT=on  OutDataTypeStr=Inherit: Same as first input
  Reshape : Reshape  OutputDimensionality=Column vector (2-D)
  Reshape1 : Reshape
  Fgrav : Outport
  wires:
  Inertial to Body/1 -> Reshape1/1
  g/1 -> Gravity in Earth Axes/1
  DCM/1 -> Inertial to Body/1
  Gravity in Earth Axes/1 -> Reshape/1
  Reshape/1 -> Inertial to Body/2
  Reshape1/1 -> Fgrav/1

== system simulator_model/Simulateur/Spitfire Airframe/Aircraft Dynamics/Total Forces  and Moments/Aerodynamics/Actuator Increments ==
  alpha : Inport
  beta : Inport  Port=2
  Actuator Deflections : Inport  Port=3
  Aileron : Subsystem
  Elevator : Subsystem
  Flap : Subsystem
  Rudder : Subsystem
  Sum : Sum  Inputs=++++  SaturateOnIntegerOverflow=on  InputSameDT=on  OutDataTypeStr=Inherit: Same as first input
  Coefficients : Outport
  wires:
  Actuator Deflections/1 -> Flap/2(Actuators), Aileron/2(Actuators), Elevator/1(Actuators), Rudder/2(Actuators)
  alpha/1 -> Flap/1(Alpha), Rudder/1(Alpha), Aileron/1(alpha)
  beta/1 -> Elevator/2(Beta)
  Aileron/1(delCoeff) -> Sum/1
  Elevator/1(delCoeff) -> Sum/2
  Rudder/1(delCoeff) -> Sum/3
  Flap/1(delCoeff) -> Sum/4
  Sum/1 -> Coefficients/1

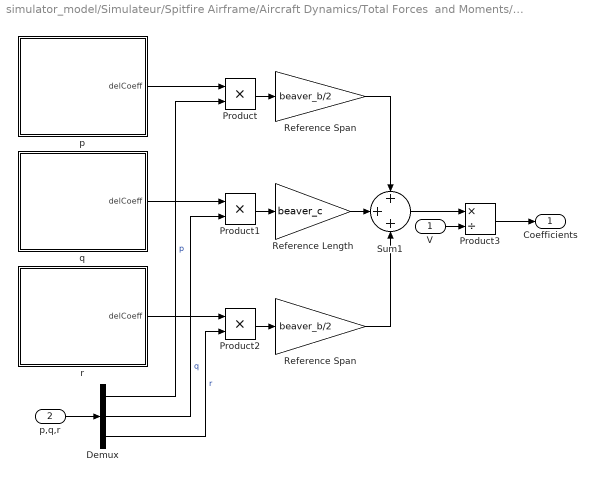
== system simulator_model/Simulateur/Spitfire Airframe/Aircraft Dynamics/Total Forces  and Moments/Aerodynamics/Body Rate Damping ==
  V : Inport
  p,q,r : Inport  Port=2
  Demux : Demux  Outputs=3
  Product : Product  SaturateOnIntegerOverflow=on  InputSameDT=on  OutDataTypeStr=Inherit: Same as first input
  Product1 : Product  SaturateOnIntegerOverflow=on  InputSameDT=on  OutDataTypeStr=Inherit: Same as first input
  Product2 : Product  SaturateOnIntegerOverflow=on  InputSameDT=on  OutDataTypeStr=Inherit: Same as first input
  Product3 : Product  Inputs=*/  SaturateOnIntegerOverflow=on  InputSameDT=on  OutDataTypeStr=Inherit: Same as first input
  Reference Length : Gain  Gain=beaver_c  SaturateOnIntegerOverflow=on  OutDataTypeStr=Inherit: Same as input  ParamDataTypeStr=Inherit: Same as input
  Reference Span : Gain  Gain=beaver_b/2  SaturateOnIntegerOverflow=on  OutDataTypeStr=Inherit: Same as input  ParamDataTypeStr=Inherit: Same as input
  "Reference Span " : Gain  Gain=beaver_b/2  SaturateOnIntegerOverflow=on  OutDataTypeStr=Inherit: Same as input  ParamDataTypeStr=Inherit: Same as input
  Sum1 : Sum  Inputs=+++  SaturateOnIntegerOverflow=on  InputSameDT=on  OutDataTypeStr=Inherit: Same as first input
  p : Subsystem
  q : Subsystem
  r : Subsystem
  Coefficients : Outport
  wires:
  p/1(delCoeff) -> Product/1
  q/1(delCoeff) -> Product1/1
  p,q,r/1 -> Demux/1
  Demux/1 -> Product/2  "p"
  Demux/2 -> Product1/2  "q"
  Demux/3 -> Product2/2  "r"
  Sum1/1 -> Product3/1
  V/1 -> Product3/2
  Product3/1 -> Coefficients/1
  Product1/1 -> Reference Length/1
  Product2/1 -> "Reference Span "/1
  Product/1 -> Reference Span/1
  r/1(delCoeff) -> Product2/1
  Reference Length/1 -> Sum1/2
  Reference Span/1 -> Sum1/1
  "Reference Span "/1 -> Sum1/3

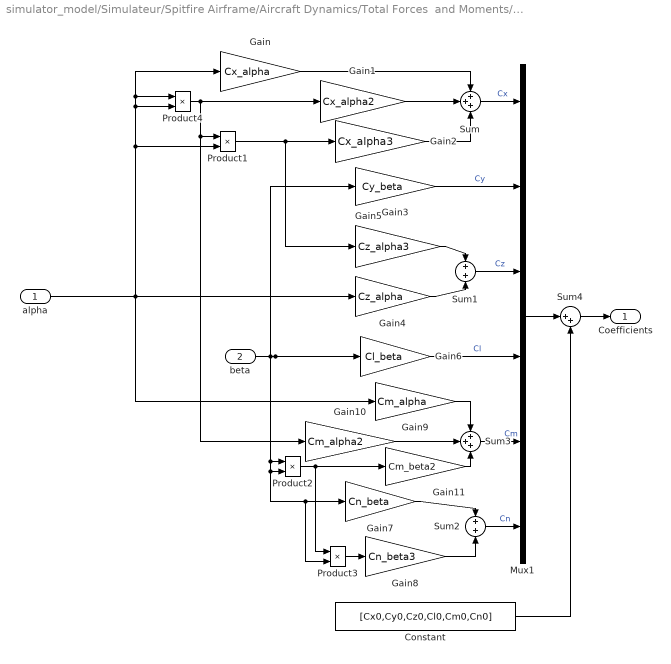
== system simulator_model/Simulateur/Spitfire Airframe/Aircraft Dynamics/Total Forces  and Moments/Aerodynamics/Datum Coefficients ==
  alpha : Inport
  beta : Inport  Port=2
  Constant : Constant  Value=[Cx0,Cy0,Cz0,Cl0,Cm0,Cn0]
  Gain : Gain  Gain=Cx_alpha  SaturateOnIntegerOverflow=on  OutDataTypeStr=Inherit: Same as input  ParamDataTypeStr=Inherit: Same as input
  Gain1 : Gain  Gain=Cx_alpha2  SaturateOnIntegerOverflow=on  OutDataTypeStr=Inherit: Same as input  ParamDataTypeStr=Inherit: Same as input
  Gain10 : Gain  Gain=Cm_alpha2  SaturateOnIntegerOverflow=on  OutDataTypeStr=Inherit: Same as input  ParamDataTypeStr=Inherit: Same as input
  Gain11 : Gain  Gain=Cm_beta2  SaturateOnIntegerOverflow=on  OutDataTypeStr=Inherit: Same as input  ParamDataTypeStr=Inherit: Same as input
  Gain2 : Gain  Gain=Cx_alpha3  SaturateOnIntegerOverflow=on  OutDataTypeStr=Inherit: Same as input  ParamDataTypeStr=Inherit: Same as input
  Gain3 : Gain  Gain=Cy_beta  SaturateOnIntegerOverflow=on  OutDataTypeStr=Inherit: Same as input  ParamDataTypeStr=Inherit: Same as input
  Gain4 : Gain  Gain=Cz_alpha  SaturateOnIntegerOverflow=on  OutDataTypeStr=Inherit: Same as input  ParamDataTypeStr=Inherit: Same as input
  Gain5 : Gain  Gain=Cz_alpha3  SaturateOnIntegerOverflow=on  OutDataTypeStr=Inherit: Same as input  ParamDataTypeStr=Inherit: Same as input
  Gain6 : Gain  Gain=Cl_beta  SaturateOnIntegerOverflow=on  OutDataTypeStr=Inherit: Same as input  ParamDataTypeStr=Inherit: Same as input
  Gain7 : Gain  Gain=Cn_beta  SaturateOnIntegerOverflow=on  OutDataTypeStr=Inherit: Same as input  ParamDataTypeStr=Inherit: Same as input
  Gain8 : Gain  Gain=Cn_beta3  SaturateOnIntegerOverflow=on  OutDataTypeStr=Inherit: Same as input  ParamDataTypeStr=Inherit: Same as input
  Gain9 : Gain  Gain=Cm_alpha  SaturateOnIntegerOverflow=on  OutDataTypeStr=Inherit: Same as input  ParamDataTypeStr=Inherit: Same as input
  Mux1 : Mux  Inputs=6
  Product{1..4} (4 alike) : Product  SaturateOnIntegerOverflow=on  InputSameDT=on  OutDataTypeStr=Inherit: Same as first input
  Sum : Sum  Inputs=+++  SaturateOnIntegerOverflow=on
  Sum1 : Sum  SaturateOnIntegerOverflow=on
  Sum2 : Sum  SaturateOnIntegerOverflow=on
  Sum3 : Sum  Inputs=+++  SaturateOnIntegerOverflow=on
  Sum4 : Sum  Inputs=|++  SaturateOnIntegerOverflow=on
  Coefficients : Outport
  wires:
  Constant/1 -> Sum4/2
  Sum4/1 -> Coefficients/1
  Mux1/1 -> Sum4/1
  Gain10/1 -> Sum3/2
  Product2/1 -> Product3/1, Gain11/1
  Gain11/1 -> Sum3/3
  Gain9/1 -> Sum3/1
  Sum3/1 -> Mux1/5  "Cm"
  Product3/1 -> Gain8/1
  Gain8/1 -> Sum2/2
  Gain7/1 -> Sum2/1
  Gain5/1 -> Sum1/1
  Gain4/1 -> Sum1/2
  Product1/1 -> Gain5/1, Gain2/1
  Gain2/1 -> Sum/3
  Product4/1 -> Product1/1, Gain10/1, Gain1/1
  Gain1/1 -> Sum/2
  Gain/1 -> Sum/1
  Sum2/1 -> Mux1/6  "Cn"
  Sum/1 -> Mux1/1  "Cx"
  Sum1/1 -> Mux1/3  "Cz"
  Gain3/1 -> Mux1/2  "Cy"
  Gain6/1 -> Mux1/4  "Cl"
  alpha/1 -> Product1/2, Product4/2, Product4/1, Gain/1, Gain9/1, Gain4/1
  beta/1 -> Gain3/1, Product3/2, Gain7/1, Product2/2, Product2/1, Gain6/1

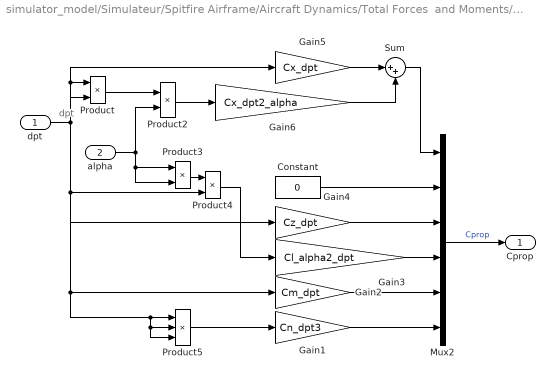
== system simulator_model/Simulateur/Spitfire Airframe/Aircraft Dynamics/Total Forces  and Moments/Engine /eng ==
  note: dpt
  dpt : Inport
  alpha : Inport  Port=2
  Constant : Constant  Value=0
  Gain1 : Gain  Gain=Cn_dpt3  SaturateOnIntegerOverflow=on  OutDataTypeStr=Inherit: Same as input  ParamDataTypeStr=Inherit: Same as input
  Gain2 : Gain  Gain=Cm_dpt  SaturateOnIntegerOverflow=on  OutDataTypeStr=Inherit: Same as input  ParamDataTypeStr=Inherit: Same as input
  Gain3 : Gain  Gain=Cl_alpha2_dpt  SaturateOnIntegerOverflow=on  OutDataTypeStr=Inherit: Same as input  ParamDataTypeStr=Inherit: Same as input
  Gain4 : Gain  Gain=Cz_dpt  SaturateOnIntegerOverflow=on  OutDataTypeStr=Inherit: Same as input  ParamDataTypeStr=Inherit: Same as input
  Gain5 : Gain  Gain=Cx_dpt  SaturateOnIntegerOverflow=on  OutDataTypeStr=Inherit: Same as input  ParamDataTypeStr=Inherit: Same as input
  Gain6 : Gain  Gain=Cx_dpt2_alpha  SaturateOnIntegerOverflow=on  OutDataTypeStr=Inherit: Same as input  ParamDataTypeStr=Inherit: Same as input
  Mux2 : Mux  Inputs=6
  Product{,2..4} (4 alike) : Product  SaturateOnIntegerOverflow=on  OutDataTypeStr=Inherit: Same as first input
  Product5 : Product  Inputs=3  SaturateOnIntegerOverflow=on  OutDataTypeStr=Inherit: Same as first input
  Sum : Sum  Inputs=|++  SaturateOnIntegerOverflow=on
  Cprop : Outport
  wires:
  Product5/1 -> Gain1/1
  Sum/1 -> Mux2/1
  Gain6/1 -> Sum/2
  Gain5/1 -> Sum/1
  Constant/1 -> Mux2/2
  Gain4/1 -> Mux2/3
  Gain3/1 -> Mux2/4
  Gain2/1 -> Mux2/5
  Gain1/1 -> Mux2/6
  Product4/1 -> Gain3/1
  Product2/1 -> Gain6/1
  dpt/1 -> Gain5/1, Product5/3, Product5/2, Product5/1, Gain2/1, Gain4/1, Product/2, Product/1, Product4/2
  alpha/1 -> Product2/2, Product3/1, Product3/2
  Mux2/1 -> Cprop/1  "Cprop"
  Product/1 -> Product2/1
  Product3/1 -> Product4/1

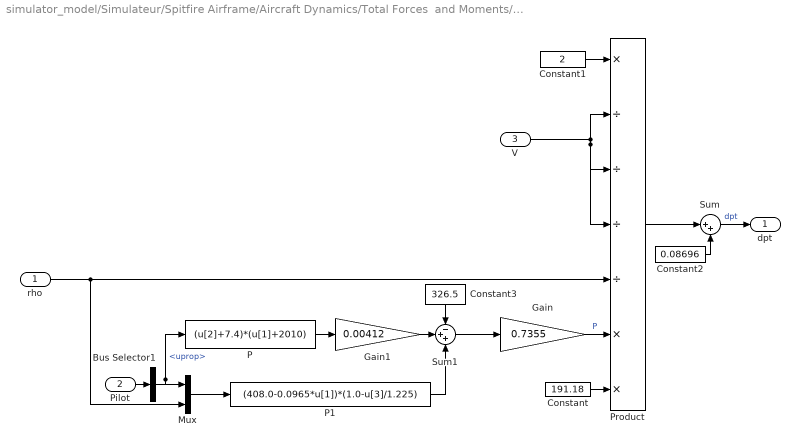
== system simulator_model/Simulateur/Spitfire Airframe/Aircraft Dynamics/Total Forces  and Moments/Engine /pow ==
  rho : Inport
  Pilot : Inport  Port=2
  V : Inport  Port=3
  Bus Selector1 : BusSelector  OutputSignals=uprop
  Constant : Constant  Value=191.18
  Constant1 : Constant  Value=2
  Constant2 : Constant  Value=0.08696
  Constant3 : Constant  Value=326.5
  Gain : Gain  Gain=0.7355  SaturateOnIntegerOverflow=on  OutDataTypeStr=Inherit: Same as input  ParamDataTypeStr=Inherit: Same as input
  Gain1 : Gain  Gain=0.00412  SaturateOnIntegerOverflow=on  OutDataTypeStr=Inherit: Same as input  ParamDataTypeStr=Inherit: Same as input
  Mux : Mux  Inputs=2
  P : Fcn  Expr=(u[2]+7.4)*(u[1]+2010)
  P1 : Fcn  Expr=(408.0-0.0965*u[1])*(1.0-u[3]/1.225)
  Product : Product  Inputs=*////**  SaturateOnIntegerOverflow=on  OutDataTypeStr=Inherit: Same as first input
  Sum : Sum  Inputs=|++  SaturateOnIntegerOverflow=on
  Sum1 : Sum  Inputs=-++  SaturateOnIntegerOverflow=on
  dpt : Outport
  wires:
  P1/1 -> Sum1/3
  Constant3/1 -> Sum1/1
  Gain1/1 -> Sum1/2
  Mux/1 -> P1/1
  Sum1/1 -> Gain/1
  P/1 -> Gain1/1
  Gain/1 -> Product/6  "P"
  rho/1 -> Mux/2, Product/5
  Sum/1 -> dpt/1  "dpt"
  V/1 -> Product/4, Product/3, Product/2
  Bus Selector1/1 -> Mux/1, P/1  "<uprop>"
  Constant/1 -> Product/7
  Constant1/1 -> Product/1
  Product/1 -> Sum/1
  Constant2/1 -> Sum/2
  Pilot/1 -> Bus Selector1/1

== system simulator_model/Simulateur/Spitfire Airframe/Aircraft Dynamics/Total Forces  and Moments/Aerodynamics/Actuator Increments/Aileron ==
  alpha : Inport
  Actuators : Inport  Port=2
  Gain1 : Gain  Gain=0  SaturateOnIntegerOverflow=on  OutDataTypeStr=Inherit: Same as input  ParamDataTypeStr=Inherit: Same as input
  Gain2 : Gain  Gain=Cy_da  SaturateOnIntegerOverflow=on  OutDataTypeStr=Inherit: Same as input  ParamDataTypeStr=Inherit: Same as input
  Gain3 : Gain  Gain=0  SaturateOnIntegerOverflow=on  OutDataTypeStr=Inherit: Same as input  ParamDataTypeStr=Inherit: Same as input
  Gain4 : Gain  Gain=Cn_da  SaturateOnIntegerOverflow=on  OutDataTypeStr=Inherit: Same as input  ParamDataTypeStr=Inherit: Same as input
  Gain5 : Gain  Gain=0  SaturateOnIntegerOverflow=on  OutDataTypeStr=Inherit: Same as input  ParamDataTypeStr=Inherit: Same as input
  Gain6 : Gain  Gain=Cl_da  SaturateOnIntegerOverflow=on  OutDataTypeStr=Inherit: Same as input  ParamDataTypeStr=Inherit: Same as input
  Gain7 : Gain  Gain=Cl_da_alpha  SaturateOnIntegerOverflow=on  OutDataTypeStr=Inherit: Same as input  ParamDataTypeStr=Inherit: Same as input
  Mux1 : Mux  Inputs=6
  Product4 : Product  SaturateOnIntegerOverflow=on  InputSameDT=on  OutDataTypeStr=Inherit: Same as first input
  Selector1 : Selector  IndexMode=Zero-based  InputPortWidth=4
  Sum1 : Sum  Inputs=++|  SaturateOnIntegerOverflow=on
  delCoeff : Outport
  wires:
  Gain6/1 -> Sum1/1
  Sum1/1 -> Mux1/4
  Gain7/1 -> Sum1/2
  Product4/1 -> Gain7/1
  Gain1/1 -> Mux1/1  "Cx"
  alpha/1 -> Product4/2
  Actuators/1 -> Selector1/1
  Mux1/1 -> delCoeff/1
  Gain2/1 -> Mux1/2  "Cy"
  Gain3/1 -> Mux1/3  "Cz"
  Gain5/1 -> Mux1/5  "Cm"
  Gain4/1 -> Mux1/6
  Selector1/1 -> Gain1/1, Gain2/1, Gain3/1, Gain6/1, Product4/1, Gain5/1, Gain4/1

== system simulator_model/Simulateur/Spitfire Airframe/Aircraft Dynamics/Total Forces  and Moments/Aerodynamics/Actuator Increments/Elevator ==
  Actuators : Inport
  Beta : Inport  Port=2
  Constant1 : Constant  Value=0
  Gain1 : Gain  Gain=Cz_de  SaturateOnIntegerOverflow=on  OutDataTypeStr=Inherit: Same as input  ParamDataTypeStr=Inherit: Same as input
  Gain2 : Gain  Gain=Cz_de_beta  SaturateOnIntegerOverflow=on  OutDataTypeStr=Inherit: Same as input  ParamDataTypeStr=Inherit: Same as input
  Gain3 : Gain  Gain=Cm_de  SaturateOnIntegerOverflow=on  OutDataTypeStr=Inherit: Same as input  ParamDataTypeStr=Inherit: Same as input
  Mux1 : Mux  Inputs=6
  Product4 : Product  Inputs=3  SaturateOnIntegerOverflow=on  InputSameDT=on  OutDataTypeStr=Inherit: Same as first input
  Selector1 : Selector  IndexMode=Zero-based  InputPortWidth=4  Indices=0
  Sum1 : Sum  SaturateOnIntegerOverflow=on
  delCoeff : Outport
  wires:
  Gain3/1 -> Mux1/5
  Gain1/1 -> Sum1/2
  Gain2/1 -> Sum1/1
  Sum1/1 -> Mux1/3
  Product4/1 -> Gain2/1
  Beta/1 -> Product4/2, Product4/1
  Mux1/1 -> delCoeff/1
  Selector1/1 -> Gain3/1, Gain1/1, Product4/3
  Constant1/1 -> Mux1/1, Mux1/2, Mux1/4, Mux1/6
  Actuators/1 -> Selector1/1

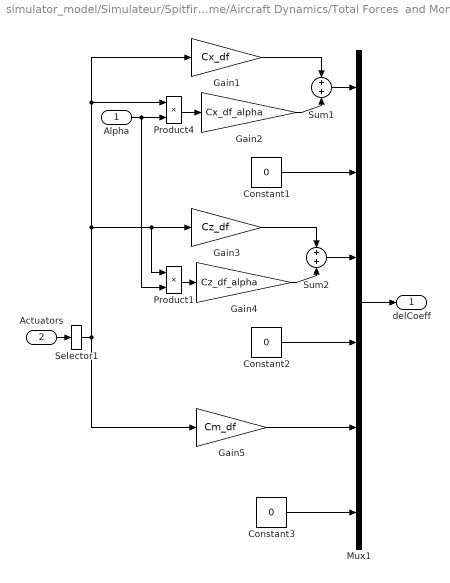
== system simulator_model/Simulateur/Spitfire Airframe/Aircraft Dynamics/Total Forces  and Moments/Aerodynamics/Actuator Increments/Flap ==
  Alpha : Inport
  Actuators : Inport  Port=2
  Constant1 : Constant  Value=0
  Constant2 : Constant  Value=0
  Constant3 : Constant  Value=0
  Gain1 : Gain  Gain=Cx_df  SaturateOnIntegerOverflow=on  OutDataTypeStr=Inherit: Same as input  ParamDataTypeStr=Inherit: Same as input
  Gain2 : Gain  Gain=Cx_df_alpha  SaturateOnIntegerOverflow=on  OutDataTypeStr=Inherit: Same as input  ParamDataTypeStr=Inherit: Same as input
  Gain3 : Gain  Gain=Cz_df  SaturateOnIntegerOverflow=on  OutDataTypeStr=Inherit: Same as input  ParamDataTypeStr=Inherit: Same as input
  Gain4 : Gain  Gain=Cz_df_alpha  SaturateOnIntegerOverflow=on  OutDataTypeStr=Inherit: Same as input  ParamDataTypeStr=Inherit: Same as input
  Gain5 : Gain  Gain=Cm_df  SaturateOnIntegerOverflow=on  OutDataTypeStr=Inherit: Same as input  ParamDataTypeStr=Inherit: Same as input
  Mux1 : Mux  Inputs=6
  Product1 : Product  SaturateOnIntegerOverflow=on  InputSameDT=on  OutDataTypeStr=Inherit: Same as first input
  Product4 : Product  SaturateOnIntegerOverflow=on  InputSameDT=on  OutDataTypeStr=Inherit: Same as first input
  Selector1 : Selector  IndexMode=Zero-based  InputPortWidth=4  Indices=3
  Sum1 : Sum  SaturateOnIntegerOverflow=on
  Sum2 : Sum  SaturateOnIntegerOverflow=on
  delCoeff : Outport
  wires:
  Selector1/1 -> Gain1/1, Product4/1, Product1/1, Gain3/1, Gain5/1
  Actuators/1 -> Selector1/1
  Gain5/1 -> Mux1/5
  Gain3/1 -> Sum2/1
  Gain4/1 -> Sum2/2
  Product1/1 -> Gain4/1
  Gain1/1 -> Sum1/1
  Gain2/1 -> Sum1/2
  Product4/1 -> Gain2/1
  Alpha/1 -> Product1/2, Product4/2
  Mux1/1 -> delCoeff/1
  Sum1/1 -> Mux1/1
  Sum2/1 -> Mux1/3
  Constant1/1 -> Mux1/2
  Constant2/1 -> Mux1/4
  Constant3/1 -> Mux1/6

== system simulator_model/Simulateur/Spitfire Airframe/Aircraft Dynamics/Total Forces  and Moments/Aerodynamics/Actuator Increments/Rudder ==
  Alpha : Inport
  Actuators : Inport  Port=2
  Constant1 : Constant  Value=0
  Constant2 : Constant  Value=0
  Gain1 : Gain  Gain=Cl_dr  SaturateOnIntegerOverflow=on  OutDataTypeStr=Inherit: Same as input  ParamDataTypeStr=Inherit: Same as input
  Gain2 : Gain  Gain=Cn_dr  SaturateOnIntegerOverflow=on  OutDataTypeStr=Inherit: Same as input  ParamDataTypeStr=Inherit: Same as input
  Gain3 : Gain  Gain=Cy_dr_alpha  SaturateOnIntegerOverflow=on  OutDataTypeStr=Inherit: Same as input  ParamDataTypeStr=Inherit: Same as input
  Gain4 : Gain  Gain=Cy_dr  SaturateOnIntegerOverflow=on  OutDataTypeStr=Inherit: Same as input  ParamDataTypeStr=Inherit: Same as input
  Gain5 : Gain  Gain=Cx_dr  SaturateOnIntegerOverflow=on  OutDataTypeStr=Inherit: Same as input  ParamDataTypeStr=Inherit: Same as input
  Mux1 : Mux  Inputs=6
  Product1 : Product  SaturateOnIntegerOverflow=on  InputSameDT=on  OutDataTypeStr=Inherit: Same as first input
  Selector1 : Selector  IndexMode=Zero-based  InputPortWidth=4  Indices=2
  Sum1 : Sum  SaturateOnIntegerOverflow=on
  delCoeff : Outport
  wires:
  Gain5/1 -> Mux1/1
  Gain4/1 -> Sum1/1
  Gain3/1 -> Sum1/2
  Gain1/1 -> Mux1/4
  Gain2/1 -> Mux1/6
  Product1/1 -> Gain3/1
  Alpha/1 -> Product1/2
  Mux1/1 -> delCoeff/1
  Actuators/1 -> Selector1/1
  Sum1/1 -> Mux1/2
  Constant1/1 -> Mux1/3
  Constant2/1 -> Mux1/5
  Selector1/1 -> Gain5/1, Gain4/1, Gain1/1, Gain2/1, Product1/1

== system simulator_model/Simulateur/Spitfire Airframe/Aircraft Dynamics/Total Forces  and Moments/Aerodynamics/Body Rate Damping/p ==
  Constant1 : Constant  Value=0
  Constant2 : Constant  Value=Cy_p
  Constant3 : Constant  Value=Cl_p
  Constant4 : Constant  Value=Cn_p
  Mux1 : Mux  Inputs=6
  delCoeff : Outport
  wires:
  Constant2/1 -> Mux1/2
  Mux1/1 -> delCoeff/1
  Constant1/1 -> Mux1/5, Mux1/3, Mux1/1
  Constant4/1 -> Mux1/6
  Constant3/1 -> Mux1/4

== system simulator_model/Simulateur/Spitfire Airframe/Aircraft Dynamics/Total Forces  and Moments/Aerodynamics/Body Rate Damping/q ==
  Constant1 : Constant  Value=0
  Constant2 : Constant  Value=Cz_q
  Constant3 : Constant  Value=Cx_q
  Constant4 : Constant  Value=Cm_q
  Constant5 : Constant  Value=Cn_q
  Mux1 : Mux  Inputs=6
  delCoeff : Outport
  wires:
  Constant2/1 -> Mux1/3
  Constant5/1 -> Mux1/6
  Constant1/1 -> Mux1/4, Mux1/2
  Constant4/1 -> Mux1/5
  Constant3/1 -> Mux1/1
  Mux1/1 -> delCoeff/1

== system simulator_model/Simulateur/Spitfire Airframe/Aircraft Dynamics/Total Forces  and Moments/Aerodynamics/Body Rate Damping/r ==
  Constant : Constant  Value=0
  Constant1 : Constant  Value=Cy_r
  Constant2 : Constant  Value=Cl_r
  Constant3 : Constant  Value=Cm_r
  Constant4 : Constant  Value=Cn_r
  Mux1 : Mux  Inputs=6
  delCoeff : Outport
  wires:
  Constant3/1 -> Mux1/5
  Constant1/1 -> Mux1/2
  Constant4/1 -> Mux1/6
  Constant2/1 -> Mux1/4
  Constant/1 -> Mux1/3, Mux1/1
  Mux1/1 -> delCoeff/1
